simulink model "Lab3Circuit2"  (R2022a)
settings: Solver=VariableStepAuto  StartTime=0.0  StopTime=10.0  RelTol=1e-3
libraries: fl_lib x15, nesl_utility x8
settings Model: Creator=bdawg  LastModifiedBy=bdawg

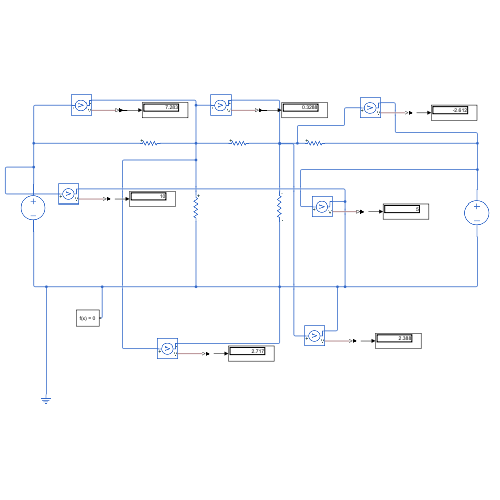
[thumbnail: Simulink's stored preview of the top-level diagram]
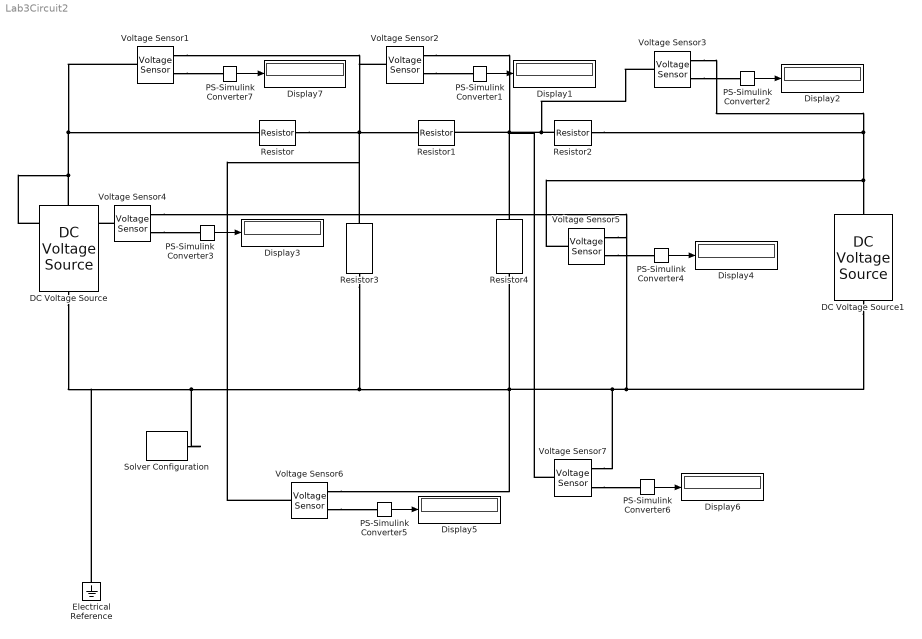
== system Lab3Circuit2 ==
  DC Voltage Source : fl_lib/Electrical/Electrical Sources/DC Voltage Source  v0=10 V
      settings: SourceProductBaseCode=PW,SS,VE
  DC Voltage Source1 : fl_lib/Electrical/Electrical Sources/DC Voltage Source  v0=5 V
      settings: SourceProductBaseCode=PW,SS,VE
  Display{1..7} (7 alike) : Display
  Electrical Reference : fl_lib/Electrical/Electrical Elements/Electrical Reference
      settings: SourceProductBaseCode=PW,SS,VE
  PS-Simulink Converter{1..7} (7 alike) : nesl_utility/PS-Simulink Converter  PhysicalDomain=network_engine_domain  SubClassName=ps_output  LeftPortType=input  RightPortType=output  PseudoPeriodic=off  Frequencies=[]  VectorFormat=inherit  Unit=inherit  AffineConversion=off
      settings: SourceProductBaseCode=SS,PW,VE
  Resistor : fl_lib/Electrical/Electrical Elements/Resistor  R=1000 Ohm  i_specify=off  i_priority=None  i=0 A  i_nominal_specify=off  i_nominal_unit=A  i_nominal_value=1  v_specify=off  v_priority=None  v=0 V  v_nominal_specify=off  v_nominal_unit=V  v_nominal_value=1
      settings: SourceProductBaseCode=PW,SS,VE
  Resistor1 : fl_lib/Electrical/Electrical Elements/Resistor  R=100 Ohm  i_specify=off  i_priority=None  i=0 A  i_nominal_specify=off  i_nominal_unit=A  i_nominal_value=1  v_specify=off  v_priority=None  v=0 V  v_nominal_specify=off  v_nominal_unit=V  v_nominal_value=1
      settings: SourceProductBaseCode=PW,SS,VE
  Resistor2 : fl_lib/Electrical/Electrical Elements/Resistor  R=470 Ohm  i_specify=off  i_priority=None  i=0 A  i_nominal_specify=off  i_nominal_unit=A  i_nominal_value=1  v_specify=off  v_priority=None  v=0 V  v_nominal_specify=off  v_nominal_unit=V  v_nominal_value=1
      settings: SourceProductBaseCode=PW,SS,VE
  Resistor3 : fl_lib/Electrical/Electrical Elements/Resistor  R=680 Ohm  i_specify=off  i_priority=None  i=0 A  i_nominal_specify=off  i_nominal_unit=A  i_nominal_value=1  v_specify=off  v_priority=None  v=0 V  v_nominal_specify=off  v_nominal_unit=V  v_nominal_value=1
      settings: SourceProductBaseCode=PW,SS,VE
  Resistor4 : fl_lib/Electrical/Electrical Elements/Resistor  R=270 Ohm  i_specify=off  i_priority=None  i=0 A  i_nominal_specify=off  i_nominal_unit=A  i_nominal_value=1  v_specify=off  v_priority=None  v=0 V  v_nominal_specify=off  v_nominal_unit=V  v_nominal_value=1
      settings: SourceProductBaseCode=PW,SS,VE
  Solver Configuration : nesl_utility/Solver Configuration  PhysicalDomain=network_engine_domain  SubClassName=solver  LeftPortType=input  RightPortType=generic  Tones=[]  Harmonics=[]  SimulateNoise=off  Profile=off  UseLocalSampling=off  EnableSwitchedLinearOptims=on  FrequencyDomain=off  UseCCode=off  RelTol=0.001  AbsTol=0.001  MinStep=1e-09  ToWorkspace=off  RevertToSquareIcSolve=off  NumHomotopyIterations=100  PhasorMode=off  PhasorModeNumHarmonics=1  IndexReductionMethod=DerivativeReplacement  DoDC=off  ResidualTolerance=1e-09  UseLocalSolver=off  LocalSolverChoice=NE_BACKWARD_EULER_ADVANCER  LocalSolverSampleTime=0.001  DoFixedCost=off  MaxNonlinIter=3  MaxModeIter=2  ComputeImpulses=off  ImpulseIterations=2  LinearAlgebra=auto  LinearAlgebraNumThread=0  EquationFormulation=NE_TIME_EF  DelaysMemoryBudget=1024  AutomaticFiltering=on  FilteringTimeConstant=0.001  PartitionStorageMethod=AS_NEEDED  PartitionMemoryBudget=1024  PartitionMethod=ROBUST
      settings: SourceProductBaseCode=SS,PW,VE
  Voltage Sensor{1..7} (7 alike) : fl_lib/Electrical/Electrical Sensors/Voltage Sensor
      settings: SourceProductBaseCode=PW,SS,VE
  wires:
  PS-Simulink Converter7/1 -> Display7/1
  PS-Simulink Converter1/1 -> Display1/1
  PS-Simulink Converter2/1 -> Display2/1
  PS-Simulink Converter3/1 -> Display3/1
  PS-Simulink Converter4/1 -> Display4/1
  PS-Simulink Converter5/1 -> Display5/1
  PS-Simulink Converter6/1 -> Display6/1
  connections:
  DC Voltage Source/LConn1 -- Voltage Sensor1/LConn1 -- Resistor/LConn1 -- Voltage Sensor4/LConn1
  Resistor/RConn1 -- Voltage Sensor6/LConn1 -- Resistor3/LConn1 -- Resistor1/LConn1 -- Voltage Sensor2/LConn1 -- Voltage Sensor1/RConn2
  Resistor2/LConn1 -- Voltage Sensor3/LConn1 -- Voltage Sensor2/RConn2 -- Voltage Sensor7/LConn1 -- Resistor4/LConn1 -- Resistor1/RConn1
  Resistor2/RConn1 -- Voltage Sensor5/LConn1 -- DC Voltage Source1/LConn1 -- Voltage Sensor3/RConn2
  DC Voltage Source1/RConn1 -- Voltage Sensor4/RConn2 -- Voltage Sensor5/RConn2 -- Voltage Sensor6/RConn2 -- Resistor4/RConn1 -- Solver Configuration/RConn1 -- Electrical Reference/LConn1 -- DC Voltage Source/RConn1 -- Resistor3/RConn1 -- Voltage Sensor7/RConn2
  Voltage Sensor1/RConn1 -- PS-Simulink Converter7/LConn1
  Voltage Sensor2/RConn1 -- PS-Simulink Converter1/LConn1
  Voltage Sensor3/RConn1 -- PS-Simulink Converter2/LConn1
  Voltage Sensor4/RConn1 -- PS-Simulink Converter3/LConn1
  Voltage Sensor5/RConn1 -- PS-Simulink Converter4/LConn1
  Voltage Sensor6/RConn1 -- PS-Simulink Converter5/LConn1
  Voltage Sensor7/RConn1 -- PS-Simulink Converter6/LConn1
